simulink model "AEB_MODEL_F"  (R2022b)
settings: Solver=VariableStepAuto  StartTime=0.0  StopTime=10.0  RelTol=1e-3
model workspace (MAT data in the model file):
  DISTANCE = 100
  MASS_OF_THE_VEHICLE = 1500
  MIN_THRESHOLD_FOR_TTCmin = 0.7
  SPEED_OF_THE_EGO_VEHICLE = 80
  SPEED_OF_THE_LEADING_VEHICLE = 0
  TTC_EMERGE = 2
  Var = 0
libraries: simulink x37, spsOnDelayLib x1
(part 2 of 2)

== system AEB_MODEL_F/AEB/AEB_SYSTEM/FULL_BRAKE/FB_SYSTEM_IN_LOOP/CALCULATIONS_WITH_RESPECT_TO_TTC ==
  DISTANCE_TO_AVOID_COLLISION : Inport
  INITIAL_SPEED : Inport  Port=2
  TTC_FB_IN : Inport  Port=3
  CAL_BRAKING_DECCELERATION : Subsystem
      settings: RTWMemSecFuncInitTerm=Inherit_from_model  RTWMemSecFuncExecute=Inherit_from_model  RTWMemSecDataConstants=Inherit_from_model  RTWMemSecDataInternal=Inherit_from_model  RTWMemSecDataParameters=Inherit_from_model
  CAL_TTC : Subsystem
      settings: RTWMemSecFuncInitTerm=Inherit_from_model  RTWMemSecFuncExecute=Inherit_from_model  RTWMemSecDataConstants=Inherit_from_model  RTWMemSecDataInternal=Inherit_from_model  RTWMemSecDataParameters=Inherit_from_model
  CAL_inital_after_decceleration_speed : Subsystem
      settings: RTWMemSecFuncInitTerm=Inherit_from_model  RTWMemSecFuncExecute=Inherit_from_model  RTWMemSecDataConstants=Inherit_from_model  RTWMemSecDataInternal=Inherit_from_model  RTWMemSecDataParameters=Inherit_from_model
  CAL_remainig_distance : Subsystem
      settings: RTWMemSecFuncInitTerm=Inherit_from_model  RTWMemSecFuncExecute=Inherit_from_model  RTWMemSecDataConstants=Inherit_from_model  RTWMemSecDataInternal=Inherit_from_model  RTWMemSecDataParameters=Inherit_from_model
  Subsystem4 : Subsystem
      settings: RTWMemSecFuncInitTerm=Inherit_from_model  RTWMemSecFuncExecute=Inherit_from_model  RTWMemSecDataConstants=Inherit_from_model  RTWMemSecDataInternal=Inherit_from_model  RTWMemSecDataParameters=Inherit_from_model
  TTC_AFTER_FULL_BRAKE : Outport
  SPEED_AFTER_DECCELERATION : Outport  Port=2
  REMAINING_DISTANCE_FOR_NEXT_BRAKING_ : Outport  Port=3
  wires:
  INITIAL_SPEED/1 -> CAL_BRAKING_DECCELERATION/1(INITIAL_SPEED), CAL_inital_after_decceleration_speed/1(INITIAL_SPEED), CAL_remainig_distance/1(INITIAL_SPEED)  "INITIAL_SPEED"
  DISTANCE_TO_AVOID_COLLISION/1 -> CAL_BRAKING_DECCELERATION/2(REMAINING_DISTANCE_AFTER_PARTIAL_BRAKING), CAL_remainig_distance/2(DISTANCE_TO_AVOID_COLLISION)  "DISTANCE_TO_AVOID_COLLISION"
  CAL_inital_after_decceleration_speed/2(SPEED_AFTER_FB_DECCELERATION) -> SPEED_AFTER_DECCELERATION/1  "SPEED_AFTER_DECCELERATION"
  CAL_inital_after_decceleration_speed/1(INITIAL_SPEED_M/S) -> CAL_TTC/1(INITIAL_SPEED_M/S)
  CAL_TTC/1(TTC_AFTER_FULL_BRAKE) -> TTC_AFTER_FULL_BRAKE/1  "TTC_AFTER_FULL_BRAKE"
  CAL_remainig_distance/1(remainig_distance) -> REMAINING_DISTANCE_FOR_NEXT_BRAKING_/1, CAL_TTC/2(SPEED_AFTER_DECCELERATION)  "REMAINING_DISTANCE_FOR_NEXT_BRAKING_"
  CAL_BRAKING_DECCELERATION/1(FB_DECCELERATION) -> CAL_remainig_distance/4(FB_DECCELERATION), CAL_inital_after_decceleration_speed/3(FULL_BRAKING_DECCELERATION)  "FB_DECCELERATION"
  Subsystem4/1(TTC_FB_OUT) -> CAL_remainig_distance/3(TTC_FB), CAL_inital_after_decceleration_speed/2(TTC_FB)  "TTC_FB"
  TTC_FB_IN/1 -> Subsystem4/1(TTC_FB_IN)  "TTC_FB_IN"

== system AEB_MODEL_F/AEB/AEB_SYSTEM/FULL_BRAKE/FB_SYSTEM_IN_LOOP/REMAINING_DISTANCE ==
  REMAINING_DISTANCE_FOR_NEXT_BRAKING_ : Inport
  NEXT_ITERATION : Inport  Port=2
  Switch4 : Switch  Criteria=u2 > Threshold  SaturateOnIntegerOverflow=off  InputSameDT=off
  Unit_Delay4 : UnitDelay  SampleTime=-1  HasFrameUpgradeWarning=on
  RATE_OF_REMAINING_DISTANCE_FOR_NEXT_BRAKING_ : Outport
  CAL__REMAINING_DISTANCE_FOR_NEXT_BRAKING_ : Outport  Port=2
  wires:
  Unit_Delay4/1 -> Switch4/2, CAL__REMAINING_DISTANCE_FOR_NEXT_BRAKING_/1
  REMAINING_DISTANCE_FOR_NEXT_BRAKING_/1 -> Switch4/3
  Switch4/1 -> Unit_Delay4/1, RATE_OF_REMAINING_DISTANCE_FOR_NEXT_BRAKING_/1
  NEXT_ITERATION/1 -> Switch4/1

== system AEB_MODEL_F/AEB/AEB_SYSTEM/FULL_BRAKE/FB_SYSTEM_IN_LOOP/SPEED ==
  note: ego_and_leading_vehicle_speed_comparison
  SPEED_AFTER_FB_DECCELERATION : Inport
  NEXT_ITERATION : Inport  Port=2
  Compare_To_Constant : simulink/Logic and Bit Operations/Compare To Constant  relop=<=  const=SPEED_OF_THE_LEADING_VEHICLE  OutDataTypeStr=boolean
      settings: RTWMemSecFuncInitTerm=Inherit_from_model  RTWMemSecFuncExecute=Inherit_from_model  RTWMemSecDataConstants=Inherit_from_model  RTWMemSecDataInternal=Inherit_from_model  RTWMemSecDataParameters=Inherit_from_model
  Constant : Constant  Value=0
  Multiply : Gain  Gain=3.6
  Switch : Switch  Criteria=u2 > Threshold  SaturateOnIntegerOverflow=off  InputSameDT=off
  Switch4 : Switch  Criteria=u2 > Threshold  SaturateOnIntegerOverflow=off  InputSameDT=off
  Unit_Delay4 : UnitDelay  SampleTime=-1  HasFrameUpgradeWarning=on
  RATE_OF _SPEED : Outport
  CAL__SPEED_AFTER_DECCELERATION : Outport  Port=2
  tag scope: comp_speed_ego_and_leading3=global
  wires:
  SPEED_AFTER_FB_DECCELERATION/1 -> Switch4/3  "SPEED_AFTER_FB_DECCELERATION"
  NEXT_ITERATION/1 -> Switch4/1  "NEXT_ITERATION"
  Unit_Delay4/1 -> CAL__SPEED_AFTER_DECCELERATION/1, Switch4/2  "CAL__SPEED_AFTER_DECCELERATION"
  Switch/1 -> RATE_OF _SPEED/1  "RATE_OF _SPEED"
  Compare_To_Constant/1 -> [comp_speed_ego_and_leading3], Switch/2
  Multiply/1 -> Compare_To_Constant/1
  Constant/1 -> Switch/1
  Switch4/1 -> Unit_Delay4/1, Switch/3, Multiply/1

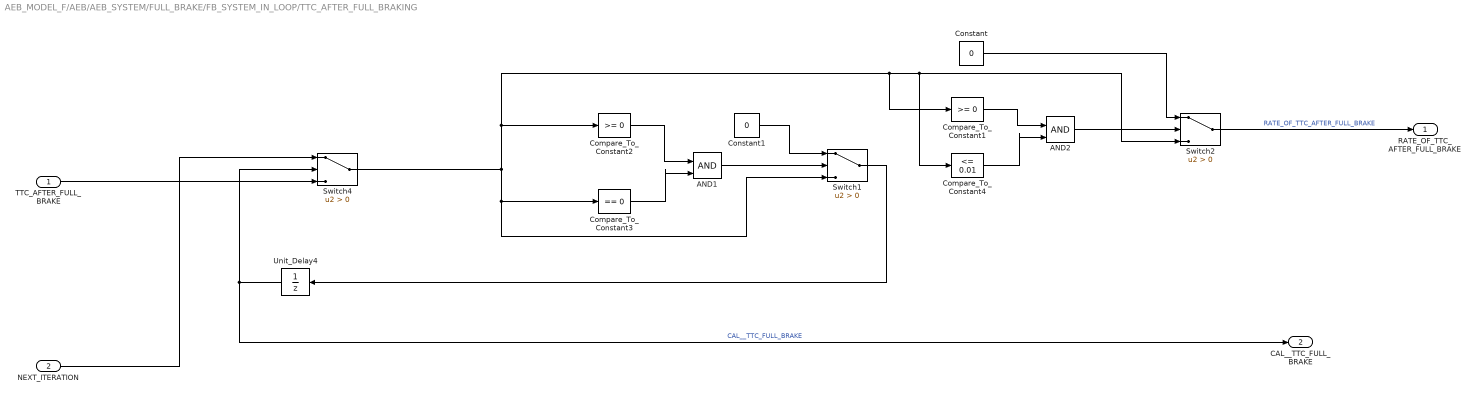
== system AEB_MODEL_F/AEB/AEB_SYSTEM/FULL_BRAKE/FB_SYSTEM_IN_LOOP/TTC_AFTER_FULL_BRAKING ==
  TTC_AFTER_FULL_BRAKE : Inport
  NEXT_ITERATION : Inport  Port=2
  AND1 : Logic  IconShape=distinctive  AllPortsSameDT=off  OutDataTypeStr=boolean
  AND2 : Logic  IconShape=distinctive  AllPortsSameDT=off  OutDataTypeStr=boolean
  Compare_To_Constant1 : simulink/Logic and Bit Operations/Compare To Constant  relop=>=  const=0  OutDataTypeStr=boolean
      settings: RTWMemSecFuncInitTerm=Inherit_from_model  RTWMemSecFuncExecute=Inherit_from_model  RTWMemSecDataConstants=Inherit_from_model  RTWMemSecDataInternal=Inherit_from_model  RTWMemSecDataParameters=Inherit_from_model
  Compare_To_Constant2 : simulink/Logic and Bit Operations/Compare To Constant  relop=>=  const=0  OutDataTypeStr=boolean
      settings: RTWMemSecFuncInitTerm=Inherit_from_model  RTWMemSecFuncExecute=Inherit_from_model  RTWMemSecDataConstants=Inherit_from_model  RTWMemSecDataInternal=Inherit_from_model  RTWMemSecDataParameters=Inherit_from_model
  Compare_To_Constant3 : simulink/Logic and Bit Operations/Compare To Constant  relop===  const=0  OutDataTypeStr=boolean
      settings: RTWMemSecFuncInitTerm=Inherit_from_model  RTWMemSecFuncExecute=Inherit_from_model  RTWMemSecDataConstants=Inherit_from_model  RTWMemSecDataInternal=Inherit_from_model  RTWMemSecDataParameters=Inherit_from_model
  Compare_To_Constant4 : simulink/Logic and Bit Operations/Compare To Constant  relop=<=  const=0.01  OutDataTypeStr=boolean
      settings: RTWMemSecFuncInitTerm=Inherit_from_model  RTWMemSecFuncExecute=Inherit_from_model  RTWMemSecDataConstants=Inherit_from_model  RTWMemSecDataInternal=Inherit_from_model  RTWMemSecDataParameters=Inherit_from_model
  Constant : Constant  Value=0
  Constant1 : Constant  Value=0
  Switch1 : Switch  Criteria=u2 > Threshold  SaturateOnIntegerOverflow=off  InputSameDT=off
  Switch2 : Switch  Criteria=u2 > Threshold  SaturateOnIntegerOverflow=off  InputSameDT=off
  Switch4 : Switch  Criteria=u2 > Threshold  SaturateOnIntegerOverflow=off  InputSameDT=off
  Unit_Delay4 : UnitDelay  SampleTime=-1  HasFrameUpgradeWarning=on
  RATE_OF_TTC_AFTER_FULL_BRAKE : Outport
  CAL__TTC_FULL_BRAKE : Outport  Port=2
  wires:
  Unit_Delay4/1 -> Switch4/2, CAL__TTC_FULL_BRAKE/1  "CAL__TTC_FULL_BRAKE"
  TTC_AFTER_FULL_BRAKE/1 -> Switch4/3
  NEXT_ITERATION/1 -> Switch4/1
  Compare_To_Constant2/1 -> AND1/1
  Compare_To_Constant3/1 -> AND1/2
  AND1/1 -> Switch1/2
  Switch1/1 -> Unit_Delay4/1
  Constant1/1 -> Switch1/1
  Switch2/1 -> RATE_OF_TTC_AFTER_FULL_BRAKE/1  "RATE_OF_TTC_AFTER_FULL_BRAKE"
  Switch4/1 -> Compare_To_Constant1/1, Switch2/3, Compare_To_Constant4/1, Compare_To_Constant2/1, Switch1/3, Compare_To_Constant3/1
  AND2/1 -> Switch2/2
  Constant/1 -> Switch2/1
  Compare_To_Constant1/1 -> AND2/1
  Compare_To_Constant4/1 -> AND2/2

== system AEB_MODEL_F/AEB/AEB_SYSTEM/PARTIAL_BRAKE/PARTIAL_BRAKING/PB_CALCULATIONS ==
  note: ego_and_leading_vehicle_speed_comparison
  note: CAL_PB
  DISTANCE_TO_AVOID_COLLISION : Inport
  INITIAL_SPEED : Inport  Port=2
  TTCmin : Inport  Port=3
  CAL_BRAKING_DECCELERATION : Subsystem
      settings: RTWMemSecFuncInitTerm=Inherit_from_model  RTWMemSecFuncExecute=Inherit_from_model  RTWMemSecDataConstants=Inherit_from_model  RTWMemSecDataInternal=Inherit_from_model  RTWMemSecDataParameters=Inherit_from_model
  CAL_INITAL_AFTER_DECCELERATION_SPEED : Subsystem
      settings: RTWMemSecFuncInitTerm=Inherit_from_model  RTWMemSecFuncExecute=Inherit_from_model  RTWMemSecDataConstants=Inherit_from_model  RTWMemSecDataInternal=Inherit_from_model  RTWMemSecDataParameters=Inherit_from_model
  CAL_REMAINING_DISTANCE : Subsystem
      settings: RTWMemSecFuncInitTerm=Inherit_from_model  RTWMemSecFuncExecute=Inherit_from_model  RTWMemSecDataConstants=Inherit_from_model  RTWMemSecDataInternal=Inherit_from_model  RTWMemSecDataParameters=Inherit_from_model
  CAL_TTC : Subsystem
      settings: RTWMemSecFuncInitTerm=Inherit_from_model  RTWMemSecFuncExecute=Inherit_from_model  RTWMemSecDataConstants=Inherit_from_model  RTWMemSecDataInternal=Inherit_from_model  RTWMemSecDataParameters=Inherit_from_model
  Compare_To_Constant : simulink/Logic and Bit Operations/Compare To Constant  relop=<=  const=SPEED_OF_THE_LEADING_VEHICLE  OutDataTypeStr=boolean
      settings: RTWMemSecFuncInitTerm=Inherit_from_model  RTWMemSecFuncExecute=Inherit_from_model  RTWMemSecDataConstants=Inherit_from_model  RTWMemSecDataInternal=Inherit_from_model  RTWMemSecDataParameters=Inherit_from_model
  Constant : Constant  Value=0
  Switch : Switch  Criteria=u2 > Threshold  SaturateOnIntegerOverflow=off  InputSameDT=off
  m/s_to_km/s : Gain  Gain=3.6
  TTC_AFTER_PARTITAL_BRAKE : Outport
  SPEED_AFTER_PB_DECCELERATION : Outport  Port=2
  REMAINING_DISTANCE_FOR_NEXT_BRAKING : Outport  Port=3
  tag scope: comp_speed_ego_and_leading_PB=global
  wires:
  CAL_BRAKING_DECCELERATION/1(PB_DECCELERATION) -> CAL_INITAL_AFTER_DECCELERATION_SPEED/3(PARTIAL_BRAKING_DECCELERATION), CAL_REMAINING_DISTANCE/4(PB_DECCELERATION)  "PB_DECCELERATION"
  INITIAL_SPEED/1 -> CAL_REMAINING_DISTANCE/1(INITIAL_SPEED), CAL_INITAL_AFTER_DECCELERATION_SPEED/1(INITIAL_SPEED)  "INITIAL_SPEED"
  TTCmin/1 -> CAL_INITAL_AFTER_DECCELERATION_SPEED/2(TTC_PB), CAL_REMAINING_DISTANCE/3(TTC_PB)  "TTCmin"
  CAL_INITAL_AFTER_DECCELERATION_SPEED/1(INITIAL_SPEED_M/S) -> CAL_TTC/1(INITIAL_SPEED_M/S)
  DISTANCE_TO_AVOID_COLLISION/1 -> CAL_BRAKING_DECCELERATION/1(DISTANCE_TO_AVOID_COLLISION), CAL_REMAINING_DISTANCE/2(DISTANCE_TO_AVOID_COLLISION)  "DISTANCE_TO_AVOID_COLLISION"
  CAL_INITAL_AFTER_DECCELERATION_SPEED/2(SPEED_AFTER_PB_DECCELERATION) -> m/s_to_km/s/1, Switch/3
  CAL_TTC/1(TTC_AFTER_PARTITAL_BRAKE) -> TTC_AFTER_PARTITAL_BRAKE/1  "TTC_AFTER_PARTITAL_BRAKE"
  CAL_REMAINING_DISTANCE/1(REMAINING_DISTANCE) -> CAL_TTC/2(SPEED_AFTER_PB_DECCELERATION), REMAINING_DISTANCE_FOR_NEXT_BRAKING/1  "REMAINING_DISTANCE_FOR_NEXT_BRAKING"
  m/s_to_km/s/1 -> Compare_To_Constant/1
  Compare_To_Constant/1 -> Switch/2, [comp_speed_ego_and_leading_PB]
  Constant/1 -> Switch/1
  Switch/1 -> SPEED_AFTER_PB_DECCELERATION/1  "SPEED_AFTER_PB_DECCELERATION"

== system AEB_MODEL_F/AEB/AEB_SYSTEM/PARTIAL_BRAKE/PARTIAL_BRAKING/PB_IN_LOOP ==
  note: condt_distance_travelled_after_brake
  TTC_AFTER_PARTITAL_BRAKE : Inport
  _SPEED_AFTER_PB_DECCELERATION : Inport  Port=2
  REMAINING_DISTANCE_FOR_NEXT_BRAKING_ : Inport  Port=3
  CALCULATIONS_WITH_RESPECT_TO_TTC : Subsystem
      settings: RTWMemSecFuncInitTerm=Inherit_from_model  RTWMemSecFuncExecute=Inherit_from_model  RTWMemSecDataConstants=Inherit_from_model  RTWMemSecDataInternal=Inherit_from_model  RTWMemSecDataParameters=Inherit_from_model
  Constant : Constant  Value=0
  REMAINING_DISTANCE : Subsystem
      settings: RTWMemSecFuncInitTerm=Inherit_from_model  RTWMemSecFuncExecute=Inherit_from_model  RTWMemSecDataConstants=Inherit_from_model  RTWMemSecDataInternal=Inherit_from_model  RTWMemSecDataParameters=Inherit_from_model
  SPEED : Subsystem
      settings: RTWMemSecFuncInitTerm=Inherit_from_model  RTWMemSecFuncExecute=Inherit_from_model  RTWMemSecDataConstants=Inherit_from_model  RTWMemSecDataInternal=Inherit_from_model  RTWMemSecDataParameters=Inherit_from_model
  Subtract : Sum  Inputs=+-
  Switch : Switch  Criteria=u2 > Threshold  SaturateOnIntegerOverflow=off  InputSameDT=off
  TTC_AFTER_PARTIAL_BRAKING : Subsystem
      settings: RTWMemSecFuncInitTerm=Inherit_from_model  RTWMemSecFuncExecute=Inherit_from_model  RTWMemSecDataConstants=Inherit_from_model  RTWMemSecDataInternal=Inherit_from_model  RTWMemSecDataParameters=Inherit_from_model
  RATE_OF_ TTC_AFTER_PARTITAL_BRAKE : Outport
  RATE_OF_SPEED : Outport  Port=2
  RATE_OF _REMAINING_DISTANCE_FOR_NEXT_BRAKING_ : Outport  Port=3
  wires:
  CALCULATIONS_WITH_RESPECT_TO_TTC/2(SPEED_AFTER_PB_DECCELERATION) -> SPEED/2(NEXT_ITERATION)  "SPEED_AFTER_PB_DECCELERATION"
  REMAINING_DISTANCE/1(RATE_OF_REMAINING_DISTANCE_FOR_NEXT_BRAKING_) -> Subtract/2, Switch/2, RATE_OF _REMAINING_DISTANCE_FOR_NEXT_BRAKING_/1  "RATE_OF _REMAINING_DISTANCE_FOR_NEXT_BRAKING_"
  CALCULATIONS_WITH_RESPECT_TO_TTC/3(REMAINING_DISTANCE_FOR_NEXT_BRAKING_) -> REMAINING_DISTANCE/2(NEXT_ITERATION)  "REMAINING_DISTANCE_FOR_NEXT_BRAKING_"
  REMAINING_DISTANCE/2(CAL__REMAINING_DISTANCE_FOR_NEXT_BRAKING_) -> CALCULATIONS_WITH_RESPECT_TO_TTC/1(DISTANCE_TO_AVOID_COLLISION)  "CAL__REMAINING_DISTANCE_FOR_NEXT_BRAKING_"
  SPEED/2(CAL__SPEED_AFTER_PB_DECCELERATION) -> CALCULATIONS_WITH_RESPECT_TO_TTC/2(INITIAL_SPEED)  "CAL__SPEED_AFTER_PB_DECCELERATION"
  SPEED/1(RATE_OF_SPEED) -> RATE_OF_SPEED/1  "RATE_OF_SPEED"
  _SPEED_AFTER_PB_DECCELERATION/1 -> SPEED/1(SPEED_AFTER_PARTITAL_BRAKE_)  "_SPEED_AFTER_PB_DECCELERATION"
  REMAINING_DISTANCE_FOR_NEXT_BRAKING_/1 -> REMAINING_DISTANCE/1(REMAINING_DISTANCE_FOR_NEXT_BRAKING _)  "REMAINING_DISTANCE_FOR_NEXT_BRAKING_"
  TTC_AFTER_PARTIAL_BRAKING/2(CAL__TTCmin) -> CALCULATIONS_WITH_RESPECT_TO_TTC/3(TTC_PB_IN)  "CAL__TTCmin"
  CALCULATIONS_WITH_RESPECT_TO_TTC/1(TTC_AFTER_PARTITAL_BRAKE) -> TTC_AFTER_PARTIAL_BRAKING/2(NEXT_ITERATION)  "TTC_AFTER_PARTITAL_BRAKE"
  TTC_AFTER_PARTITAL_BRAKE/1 -> TTC_AFTER_PARTIAL_BRAKING/1(TTC_AFTER_PARTITAL_BRAKE)  "TTC_AFTER_PARTITAL_BRAKE"
  Constant/1 -> Switch/3
  TTC_AFTER_PARTIAL_BRAKING/1(RATE_OF_TTC_AFTER_PARTITAL_BRAKE) -> RATE_OF_ TTC_AFTER_PARTITAL_BRAKE/1  "RATE_OF_ TTC_AFTER_PARTITAL_BRAKE"
  Subtract/1 -> Switch/1
  [DISTANCE_TO_AVOID_COLLISION] -> Subtract/1
  Switch/1 -> ?  "PARTIAL_BRAKE_DISTANCE_TRAVELLED_"

== system AEB_MODEL_F/AEB/BRAKE_PEDAL_FORCE_and_DIAGNOSTIC_CHECKS/BRAKE_PEDAL_FORCE_CALCULATION/COMPARING_THE_BOTH_BRAKING_DECCELERATION_VALUES/CAL.KM//Hr_TO_M//Hr_and_DISTANCE_TO_AVOID_COLLISION ==
  note: CONDITION_FOR_CHECKING_REACTION_TIME
  note: condt_TTC>5;_AEB_OFF
  INITIAL_SPEED : Inport
  DISTANCE : Inport  Port=2
  CAL_TTC : Constant  Value=DISTANCE/(SPEED_OF_THE_EGO_VEHICLE-SPEED_OF_THE_LEADING_VEHICLE)*3.6
  Compare_To_Constant : simulink/Logic and Bit Operations/Compare To Constant  relop=<  const=5  OutDataTypeStr=boolean
      settings: RTWMemSecFuncInitTerm=Inherit_from_model  RTWMemSecFuncExecute=Inherit_from_model  RTWMemSecDataConstants=Inherit_from_model  RTWMemSecDataInternal=Inherit_from_model  RTWMemSecDataParameters=Inherit_from_model
  Constant : Constant  Value=0
  Constant1 : Constant
  Divide : Product  Inputs=*/
  KM/HR_TO_M/S : Constant  Value=3.6
  Subtract : Sum  Inputs=+-
  Subtract1 : Sum  Inputs=+-
  Switch : Switch  Criteria=u2 > Threshold  SaturateOnIntegerOverflow=off  InputSameDT=off
  INITIAL_SPEED_M/S : Outport
  DISTANCE_TO_AVOID_COLLISION : Outport  Port=2
  wires:
  Subtract/1 -> Subtract1/1  "REACTION_DISTANCE"
  Constant1/1 -> Subtract1/2
  Divide/1 -> INITIAL_SPEED_M/S/1, Switch/3  "INITIAL_SPEED_M/S"
  Switch/1 -> Subtract/2  "condt_TTC<5"
  Subtract1/1 -> DISTANCE_TO_AVOID_COLLISION/1  "DISTANCE_TO_AVOID_COLLISION"
  INITIAL_SPEED/1 -> Divide/1  "SPEED"
  DISTANCE/1 -> Subtract/1  "DISTANCE"
  Compare_To_Constant/1 -> Switch/2
  KM/HR_TO_M/S/1 -> Divide/2
  CAL_TTC/1 -> Compare_To_Constant/1  "CAL_TTC"
  Constant/1 -> Switch/1

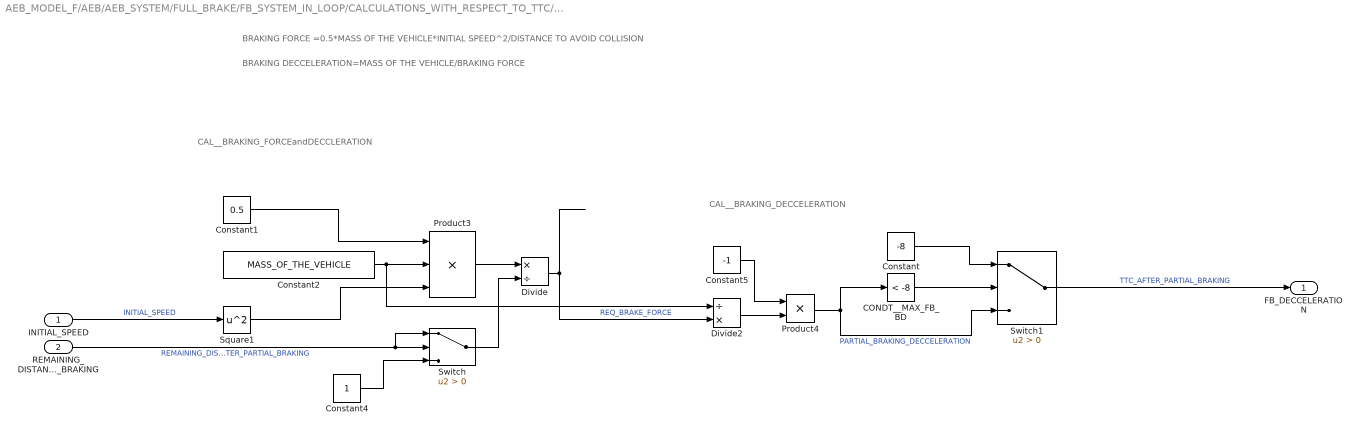
== system AEB_MODEL_F/AEB/AEB_SYSTEM/FULL_BRAKE/FB_SYSTEM_IN_LOOP/CALCULATIONS_WITH_RESPECT_TO_TTC/CAL_BRAKING_DECCELERATION ==
  note: BRAKING DECCELERATION=MASS OF THE VEHICLE/BRAKING FORCE
  note: BRAKING FORCE =0.5*MASS OF THE VEHICLE*INITIAL SPEED^2/DISTANCE TO AVOID COLLISION
  note: CAL__BRAKING_DECCELERATION
  note: CAL__BRAKING_FORCEandDECCLERATION
  INITIAL_SPEED : Inport
  REMAINING_DISTANCE_AFTER_PARTIAL_BRAKING : Inport  Port=2
  CONDT__MAX_FB_BD : simulink/Logic and Bit Operations/Compare To Constant  relop=<  const=-8  OutDataTypeStr=boolean
      settings: RTWMemSecFuncInitTerm=Inherit_from_model  RTWMemSecFuncExecute=Inherit_from_model  RTWMemSecDataConstants=Inherit_from_model  RTWMemSecDataInternal=Inherit_from_model  RTWMemSecDataParameters=Inherit_from_model
  Constant : Constant  Value=-8
  Constant1 : Constant  Value=0.5
  Constant2 : Constant  Value=MASS_OF_THE_VEHICLE
  Constant4 : Constant
  Constant5 : Constant  Value=-1
  Divide : Product  Inputs=*/
  Divide2 : Product  Inputs=/*
  Product3 : Product  Inputs=3
  Product4 : Product
  Square1 : Math  Operator=square
  Switch : Switch  Criteria=u2 > Threshold  SaturateOnIntegerOverflow=off  InputSameDT=off
  Switch1 : Switch  Criteria=u2 > Threshold  SaturateOnIntegerOverflow=off  InputSameDT=off
  FB_DECCELERATION : Outport
  wires:
  CONDT__MAX_FB_BD/1 -> Switch1/2
  Constant/1 -> Switch1/1
  INITIAL_SPEED/1 -> Square1/1  "INITIAL_SPEED"
  Constant4/1 -> Switch/3
  Switch/1 -> Divide/2
  Divide2/1 -> Product4/2
  Constant2/1 -> Divide2/1, Product3/2
  Product3/1 -> Divide/1
  REMAINING_DISTANCE_AFTER_PARTIAL_BRAKING/1 -> Switch/1, Switch/2  "REMAINING_DISTANCE_AFTER_PARTIAL_BRAKING"
  Constant5/1 -> Product4/1
  Switch1/1 -> FB_DECCELERATION/1  "TTC_AFTER_PARTIAL_BRAKING"
  Square1/1 -> Product3/3
  Product4/1 -> Switch1/3, CONDT__MAX_FB_BD/1  "PARTIAL_BRAKING_DECCELERATION"
  Divide/1 -> Divide2/2  "REQ_BRAKE_FORCE"
  Constant1/1 -> Product3/1

== system AEB_MODEL_F/AEB/AEB_SYSTEM/FULL_BRAKE/FB_SYSTEM_IN_LOOP/CALCULATIONS_WITH_RESPECT_TO_TTC/CAL_TTC ==
  INITIAL_SPEED_M/S : Inport
  SPEED_AFTER_DECCELERATION : Inport  Port=2
  Constant6 : Constant
  Divide1 : Product  Inputs=/*
  Switch2 : Switch  Criteria=u2 > Threshold  SaturateOnIntegerOverflow=off  InputSameDT=off
  TTC_AFTER_FULL_BRAKE : Outport
  wires:
  Constant6/1 -> Switch2/3
  Switch2/1 -> Divide1/1
  INITIAL_SPEED_M/S/1 -> Switch2/2, Switch2/1  "INITIAL_SPEED_M/S"
  SPEED_AFTER_DECCELERATION/1 -> Divide1/2  "SPEED_AFTER_DECCELERATION"
  Divide1/1 -> TTC_AFTER_FULL_BRAKE/1  "TTC_AFTER_FULL_BRAKE"

== system AEB_MODEL_F/AEB/AEB_SYSTEM/FULL_BRAKE/FB_SYSTEM_IN_LOOP/CALCULATIONS_WITH_RESPECT_TO_TTC/CAL_inital_after_decceleration_speed ==
  note: Speed after deceleration:
      | V = u + at
  INITIAL_SPEED : Inport
  TTC_FB : Inport  Port=2
  FULL_BRAKING_DECCELERATION : Inport  Port=3
  Product5 : Product
  Subtract1 : Sum
  INITIAL_SPEED_M/S : Outport
  SPEED_AFTER_FB_DECCELERATION : Outport  Port=2
  wires:
  INITIAL_SPEED/1 -> Subtract1/1  "INITIAL_SPEED"
  FULL_BRAKING_DECCELERATION/1 -> Product5/1  "FULL_BRAKING_DECCELERATION"
  Product5/1 -> Subtract1/2
  Subtract1/1 -> SPEED_AFTER_FB_DECCELERATION/1, INITIAL_SPEED_M/S/1  "INITIAL_SPEED_M/S"
  TTC_FB/1 -> Product5/2  "TTC_FB"

== system AEB_MODEL_F/AEB/AEB_SYSTEM/FULL_BRAKE/FB_SYSTEM_IN_LOOP/CALCULATIONS_WITH_RESPECT_TO_TTC/CAL_remainig_distance ==
  note: Remaining distance= ut + 1/2(at^2)
  INITIAL_SPEED : Inport
  DISTANCE_TO_AVOID_COLLISION : Inport  Port=2
  TTC_FB : Inport  Port=3
  FB_DECCELERATION : Inport  Port=4
  Add1 : Sum
  Constant3 : Constant  Value=0.5
  Product1 : Product  Inputs=3
  Product2 : Product
  Square2 : Math  Operator=square
  Subtract3 : Sum  Inputs=+-
  remainig_distance : Outport
  wires:
  Add1/1 -> Subtract3/2
  TTC_FB/1 -> Square2/1, Product2/2  "TTC_FB"
  Square2/1 -> Product1/3
  Subtract3/1 -> remainig_distance/1  "remainig_distance"
  Product1/1 -> Add1/2
  Product2/1 -> Add1/1
  Constant3/1 -> Product1/1
  FB_DECCELERATION/1 -> Product1/2  "FB_DECCELERATION"
  DISTANCE_TO_AVOID_COLLISION/1 -> Subtract3/1  "DISTANCE_TO_AVOID_COLLISION"
  INITIAL_SPEED/1 -> Product2/1  "INITIAL_SPEED"

== system AEB_MODEL_F/AEB/AEB_SYSTEM/FULL_BRAKE/FB_SYSTEM_IN_LOOP/CALCULATIONS_WITH_RESPECT_TO_TTC/Subsystem4 ==
  TTC_FB_IN : Inport
  AND1 : Logic  IconShape=distinctive  AllPortsSameDT=off  OutDataTypeStr=boolean
  Compare_To_Constant2 : simulink/Logic and Bit Operations/Compare To Constant  relop=<=  const=0.03  OutDataTypeStr=boolean
      settings: RTWMemSecFuncInitTerm=Inherit_from_model  RTWMemSecFuncExecute=Inherit_from_model  RTWMemSecDataConstants=Inherit_from_model  RTWMemSecDataInternal=Inherit_from_model  RTWMemSecDataParameters=Inherit_from_model
  Compare_To_Constant3 : simulink/Logic and Bit Operations/Compare To Constant  relop=>  const=0  OutDataTypeStr=boolean
      settings: RTWMemSecFuncInitTerm=Inherit_from_model  RTWMemSecFuncExecute=Inherit_from_model  RTWMemSecDataConstants=Inherit_from_model  RTWMemSecDataInternal=Inherit_from_model  RTWMemSecDataParameters=Inherit_from_model
  Constant : Constant  Value=0
  Switch1 : Switch  Criteria=u2 > Threshold  SaturateOnIntegerOverflow=off  InputSameDT=off
  TTC_FB_OUT : Outport
  wires:
  AND1/1 -> Switch1/2
  Compare_To_Constant3/1 -> AND1/2
  Compare_To_Constant2/1 -> AND1/1
  TTC_FB_IN/1 -> Compare_To_Constant2/1, Switch1/3, Compare_To_Constant3/1
  Switch1/1 -> TTC_FB_OUT/1
  Constant/1 -> Switch1/1

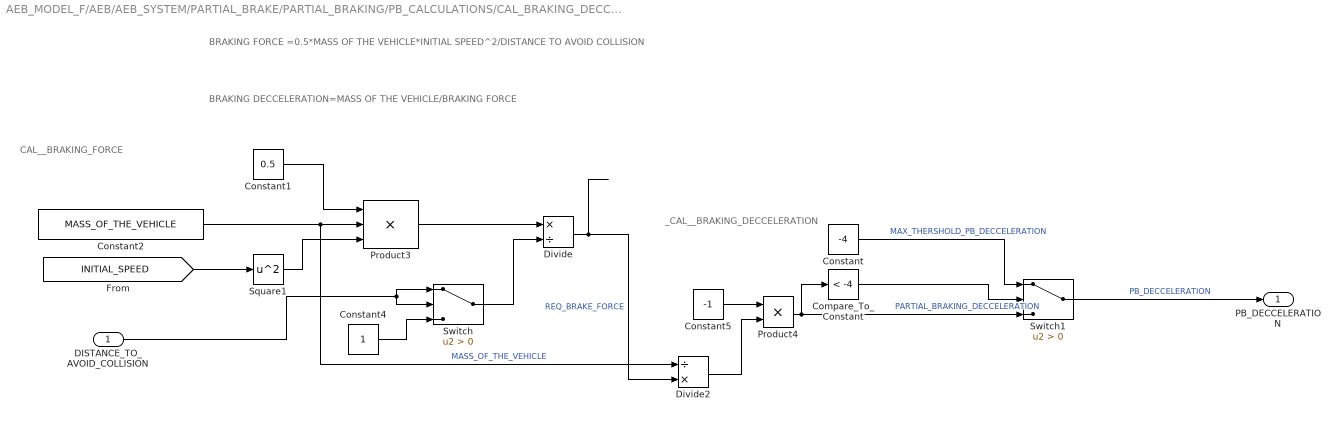
== system AEB_MODEL_F/AEB/AEB_SYSTEM/PARTIAL_BRAKE/PARTIAL_BRAKING/PB_CALCULATIONS/CAL_BRAKING_DECCELERATION ==
  note: _CAL__BRAKING_DECCELERATION
  note: CAL__BRAKING_FORCE
  note: BRAKING FORCE =0.5*MASS OF THE VEHICLE*INITIAL SPEED^2/DISTANCE TO AVOID COLLISION
  note: BRAKING DECCELERATION=MASS OF THE VEHICLE/BRAKING FORCE
  DISTANCE_TO_AVOID_COLLISION : Inport
  Compare_To_Constant : simulink/Logic and Bit Operations/Compare To Constant  relop=<  const=-4  OutDataTypeStr=boolean
      settings: RTWMemSecFuncInitTerm=Inherit_from_model  RTWMemSecFuncExecute=Inherit_from_model  RTWMemSecDataConstants=Inherit_from_model  RTWMemSecDataInternal=Inherit_from_model  RTWMemSecDataParameters=Inherit_from_model
  Constant : Constant  Value=-4
  Constant1 : Constant  Value=0.5
  Constant2 : Constant  Value=MASS_OF_THE_VEHICLE
  Constant4 : Constant
  Constant5 : Constant  Value=-1
  Divide : Product  Inputs=*/
  Divide2 : Product  Inputs=/*
  Product3 : Product  Inputs=3
  Product4 : Product
  Square1 : Math  Operator=square
  Switch : Switch  Criteria=u2 > Threshold  SaturateOnIntegerOverflow=off  InputSameDT=off
  Switch1 : Switch  Criteria=u2 > Threshold  SaturateOnIntegerOverflow=off  InputSameDT=off
  PB_DECCELERATION : Outport
  wires:
  DISTANCE_TO_AVOID_COLLISION/1 -> Switch/2, Switch/1
  Divide2/1 -> Product4/2
  Constant2/1 -> Divide2/1, Product3/2  "MASS_OF_THE_VEHICLE"
  Product4/1 -> Switch1/3, Compare_To_Constant/1  "PARTIAL_BRAKING_DECCELERATION"
  Constant1/1 -> Product3/1
  Divide/1 -> Divide2/2  "REQ_BRAKE_FORCE"
  Constant4/1 -> Switch/3
  Square1/1 -> Product3/3
  Product3/1 -> Divide/1
  Switch/1 -> Divide/2
  [INITIAL_SPEED] -> Square1/1
  Constant5/1 -> Product4/1
  Constant/1 -> Switch1/1  "MAX_THERSHOLD_PB_DECCELERATION"
  Switch1/1 -> PB_DECCELERATION/1  "PB_DECCELERATION"
  Compare_To_Constant/1 -> Switch1/2

== system AEB_MODEL_F/AEB/AEB_SYSTEM/PARTIAL_BRAKE/PARTIAL_BRAKING/PB_CALCULATIONS/CAL_INITAL_AFTER_DECCELERATION_SPEED ==
  note: Speed after deceleration:
      | V = u + at
  INITIAL_SPEED : Inport
  TTC_PB : Inport  Port=2
  PARTIAL_BRAKING_DECCELERATION : Inport  Port=3
  Product5 : Product
  Subtract1 : Sum
  INITIAL_SPEED_M/S : Outport
  SPEED_AFTER_PB_DECCELERATION : Outport  Port=2
  wires:
  INITIAL_SPEED/1 -> Subtract1/1  "INITIAL_SPEED"
  PARTIAL_BRAKING_DECCELERATION/1 -> Product5/1  "PARTIAL_BRAKING_DECCELERATION"
  Product5/1 -> Subtract1/2
  Subtract1/1 -> SPEED_AFTER_PB_DECCELERATION/1, INITIAL_SPEED_M/S/1  "INITIAL_SPEED_M/S"
  TTC_PB/1 -> Product5/2  "TTC_PB"

== system AEB_MODEL_F/AEB/AEB_SYSTEM/PARTIAL_BRAKE/PARTIAL_BRAKING/PB_CALCULATIONS/CAL_REMAINING_DISTANCE ==
  note: Remaining distance= ut + 1/2(at^2)
  INITIAL_SPEED : Inport
  DISTANCE_TO_AVOID_COLLISION : Inport  Port=2
  TTC_PB : Inport  Port=3
  PB_DECCELERATION : Inport  Port=4
  Add1 : Sum
  Constant3 : Constant  Value=0.5
  Product1 : Product  Inputs=3
  Product2 : Product
  Square2 : Math  Operator=square
  Subtract3 : Sum  Inputs=+-
  REMAINING_DISTANCE : Outport
  wires:
  Add1/1 -> Subtract3/2
  TTC_PB/1 -> Square2/1, Product2/2  "TTC_PB"
  Square2/1 -> Product1/3
  Subtract3/1 -> REMAINING_DISTANCE/1  "REMAINING_DISTANCE"
  Product1/1 -> Add1/2
  Product2/1 -> Add1/1
  Constant3/1 -> Product1/1
  PB_DECCELERATION/1 -> Product1/2  "PB_DECCELERATION"
  DISTANCE_TO_AVOID_COLLISION/1 -> Subtract3/1  "DISTANCE_TO_AVOID_COLLISION"
  INITIAL_SPEED/1 -> Product2/1  "INITIAL_SPEED"

== system AEB_MODEL_F/AEB/AEB_SYSTEM/PARTIAL_BRAKE/PARTIAL_BRAKING/PB_CALCULATIONS/CAL_TTC ==
  INITIAL_SPEED_M/S : Inport
  SPEED_AFTER_PB_DECCELERATION : Inport  Port=2
  Constant6 : Constant
  Divide1 : Product  Inputs=/*
  Switch2 : Switch  Criteria=u2 > Threshold  SaturateOnIntegerOverflow=off  InputSameDT=off
  TTC_AFTER_PARTITAL_BRAKE : Outport
  wires:
  Constant6/1 -> Switch2/3
  Switch2/1 -> Divide1/1
  INITIAL_SPEED_M/S/1 -> Switch2/2, Switch2/1  "INITIAL_SPEED_M/S"
  SPEED_AFTER_PB_DECCELERATION/1 -> Divide1/2  "SPEED_AFTER_PB_DECCELERATION"
  Divide1/1 -> TTC_AFTER_PARTITAL_BRAKE/1  "TTC_AFTER_PARTITAL_BRAKE"

== system AEB_MODEL_F/AEB/AEB_SYSTEM/PARTIAL_BRAKE/PARTIAL_BRAKING/PB_IN_LOOP/CALCULATIONS_WITH_RESPECT_TO_TTC ==
  DISTANCE_TO_AVOID_COLLISION : Inport
  INITIAL_SPEED : Inport  Port=2
  TTC_PB_IN : Inport  Port=3
  CAL_BRAKING_DECCELERATION : Subsystem
      settings: RTWMemSecFuncInitTerm=Inherit_from_model  RTWMemSecFuncExecute=Inherit_from_model  RTWMemSecDataConstants=Inherit_from_model  RTWMemSecDataInternal=Inherit_from_model  RTWMemSecDataParameters=Inherit_from_model
  CAL_TTC : Subsystem
      settings: RTWMemSecFuncInitTerm=Inherit_from_model  RTWMemSecFuncExecute=Inherit_from_model  RTWMemSecDataConstants=Inherit_from_model  RTWMemSecDataInternal=Inherit_from_model  RTWMemSecDataParameters=Inherit_from_model
  CAL_inital_after_decceleration_speed : Subsystem
      settings: RTWMemSecFuncInitTerm=Inherit_from_model  RTWMemSecFuncExecute=Inherit_from_model  RTWMemSecDataConstants=Inherit_from_model  RTWMemSecDataInternal=Inherit_from_model  RTWMemSecDataParameters=Inherit_from_model
  CAL_remainig_distance : Subsystem
      settings: RTWMemSecFuncInitTerm=Inherit_from_model  RTWMemSecFuncExecute=Inherit_from_model  RTWMemSecDataConstants=Inherit_from_model  RTWMemSecDataInternal=Inherit_from_model  RTWMemSecDataParameters=Inherit_from_model
  TTC_LIMIT : Subsystem
      settings: RTWMemSecFuncInitTerm=Inherit_from_model  RTWMemSecFuncExecute=Inherit_from_model  RTWMemSecDataConstants=Inherit_from_model  RTWMemSecDataInternal=Inherit_from_model  RTWMemSecDataParameters=Inherit_from_model
  TTC_AFTER_PARTITAL_BRAKE : Outport
  SPEED_AFTER_PB_DECCELERATION : Outport  Port=2
  REMAINING_DISTANCE_FOR_NEXT_BRAKING_ : Outport  Port=3
  wires:
  INITIAL_SPEED/1 -> CAL_BRAKING_DECCELERATION/1(INITIAL_SPEED), CAL_inital_after_decceleration_speed/1(INITIAL_SPEED), CAL_remainig_distance/1(INITIAL_SPEED)  "INITIAL_SPEED"
  DISTANCE_TO_AVOID_COLLISION/1 -> CAL_BRAKING_DECCELERATION/2(DISTANCE_TO_AVOID_COLLISION), CAL_remainig_distance/2(DISTANCE_TO_AVOID_COLLISION)  "DISTANCE_TO_AVOID_COLLISION"
  CAL_inital_after_decceleration_speed/2(SPEED_AFTER_PB_DECCELERATION) -> SPEED_AFTER_PB_DECCELERATION/1  "SPEED_AFTER_PB_DECCELERATION"
  CAL_inital_after_decceleration_speed/1(INITIAL_SPEED_M/S) -> CAL_TTC/1(INITIAL_SPEED_M/S)  "INITIAL_SPEED"
  CAL_TTC/1(TTC_AFTER_PARTITAL_BRAKE) -> TTC_AFTER_PARTITAL_BRAKE/1  "TTC_AFTER_PARTITAL_BRAKE"
  CAL_remainig_distance/1(Remainig_distance) -> CAL_TTC/2(SPEED_AFTER_PB_DECCELERATION), REMAINING_DISTANCE_FOR_NEXT_BRAKING_/1  "Remainig_distance"
  CAL_BRAKING_DECCELERATION/1(PB_DECCELERATION) -> CAL_remainig_distance/4(PB_DECCELERATION), CAL_inital_after_decceleration_speed/3(PARTIAL_BRAKING_DECCELERATION)  "PB_DECCELERATION"
  TTC_LIMIT/1(TTC_PB) -> CAL_inital_after_decceleration_speed/2(TTC_PB), CAL_remainig_distance/3(TTC_PB)  "TTC_PB"
  TTC_PB_IN/1 -> TTC_LIMIT/1(TTC_PB_)  "TTC_PB_IN"

== system AEB_MODEL_F/AEB/AEB_SYSTEM/PARTIAL_BRAKE/PARTIAL_BRAKING/PB_IN_LOOP/REMAINING_DISTANCE ==
  REMAINING_DISTANCE_FOR_NEXT_BRAKING _ : Inport
  NEXT_ITERATION : Inport  Port=2
  Switch4 : Switch  Criteria=u2 > Threshold  SaturateOnIntegerOverflow=off  InputSameDT=off
  Unit_Delay4 : UnitDelay  SampleTime=-1  HasFrameUpgradeWarning=on
  RATE_OF_REMAINING_DISTANCE_FOR_NEXT_BRAKING_ : Outport
  CAL__REMAINING_DISTANCE_FOR_NEXT_BRAKING_ : Outport  Port=2
  wires:
  REMAINING_DISTANCE_FOR_NEXT_BRAKING _/1 -> Switch4/3  "REMAINING_DISTANCE_FOR_NEXT_BRAKING _"
  Switch4/1 -> RATE_OF_REMAINING_DISTANCE_FOR_NEXT_BRAKING_/1, Unit_Delay4/1  "RATE_OF_REMAINING_DISTANCE_FOR_NEXT_BRAKING_"
  NEXT_ITERATION/1 -> Switch4/1  "NEXT_ITERATION"
  Unit_Delay4/1 -> Switch4/2, CAL__REMAINING_DISTANCE_FOR_NEXT_BRAKING_/1  "CAL__REMAINING_DISTANCE_FOR_NEXT_BRAKING_"

== system AEB_MODEL_F/AEB/AEB_SYSTEM/PARTIAL_BRAKE/PARTIAL_BRAKING/PB_IN_LOOP/SPEED ==
  note: ego_and_leading_vehicle_speed_comparison
  SPEED_AFTER_PARTITAL_BRAKE_ : Inport
  NEXT_ITERATION : Inport  Port=2
  Comp_speed_with_ego_vehicle : simulink/Logic and Bit Operations/Compare To Constant  relop=<=  const=SPEED_OF_THE_LEADING_VEHICLE  OutDataTypeStr=boolean
      settings: RTWMemSecFuncInitTerm=Inherit_from_model  RTWMemSecFuncExecute=Inherit_from_model  RTWMemSecDataConstants=Inherit_from_model  RTWMemSecDataInternal=Inherit_from_model  RTWMemSecDataParameters=Inherit_from_model
  Constant : Constant  Value=0
  Multiply : Gain  Gain=3.6
  Switch : Switch  Criteria=u2 > Threshold  SaturateOnIntegerOverflow=off  InputSameDT=off
  Switch4 : Switch  Criteria=u2 > Threshold  SaturateOnIntegerOverflow=off  InputSameDT=off
  Unit_Delay4 : UnitDelay  SampleTime=-1  HasFrameUpgradeWarning=on
  RATE_OF_SPEED : Outport
  CAL__SPEED_AFTER_PB_DECCELERATION : Outport  Port=2
  tag scope: comp_speed_ego_and_leading_pb=global
  wires:
  Unit_Delay4/1 -> Switch4/2, CAL__SPEED_AFTER_PB_DECCELERATION/1  "CAL__SPEED_AFTER_PB_DECCELERATION"
  SPEED_AFTER_PARTITAL_BRAKE_/1 -> Switch4/3  "SPEED_AFTER_PARTITAL_BRAKE_"
  NEXT_ITERATION/1 -> Switch4/1  "NEXT_ITERATION"
  Switch/1 -> RATE_OF_SPEED/1  "RATE_OF_SPEED"
  Comp_speed_with_ego_vehicle/1 -> Switch/2, [comp_speed_ego_and_leading_pb]
  Multiply/1 -> Comp_speed_with_ego_vehicle/1
  Constant/1 -> Switch/1
  Switch4/1 -> Unit_Delay4/1, Switch/3, Multiply/1

== system AEB_MODEL_F/AEB/AEB_SYSTEM/PARTIAL_BRAKE/PARTIAL_BRAKING/PB_IN_LOOP/TTC_AFTER_PARTIAL_BRAKING ==
  TTC_AFTER_PARTITAL_BRAKE : Inport
  NEXT_ITERATION : Inport  Port=2
  AND1 : Logic  IconShape=distinctive  AllPortsSameDT=off  OutDataTypeStr=boolean
  AND2 : Logic  IconShape=distinctive  AllPortsSameDT=off  OutDataTypeStr=boolean
  Compare_To_Constant1 : simulink/Logic and Bit Operations/Compare To Constant  relop=>=  const=0  OutDataTypeStr=boolean
      settings: RTWMemSecFuncInitTerm=Inherit_from_model  RTWMemSecFuncExecute=Inherit_from_model  RTWMemSecDataConstants=Inherit_from_model  RTWMemSecDataInternal=Inherit_from_model  RTWMemSecDataParameters=Inherit_from_model
  Compare_To_Constant2 : simulink/Logic and Bit Operations/Compare To Constant  relop=>=  const=0  OutDataTypeStr=boolean
      settings: RTWMemSecFuncInitTerm=Inherit_from_model  RTWMemSecFuncExecute=Inherit_from_model  RTWMemSecDataConstants=Inherit_from_model  RTWMemSecDataInternal=Inherit_from_model  RTWMemSecDataParameters=Inherit_from_model
  Compare_To_Constant3 : simulink/Logic and Bit Operations/Compare To Constant  relop===  const=0  OutDataTypeStr=boolean
      settings: RTWMemSecFuncInitTerm=Inherit_from_model  RTWMemSecFuncExecute=Inherit_from_model  RTWMemSecDataConstants=Inherit_from_model  RTWMemSecDataInternal=Inherit_from_model  RTWMemSecDataParameters=Inherit_from_model
  Compare_To_Constant4 : simulink/Logic and Bit Operations/Compare To Constant  relop=<=  const=0.01  OutDataTypeStr=boolean
      settings: RTWMemSecFuncInitTerm=Inherit_from_model  RTWMemSecFuncExecute=Inherit_from_model  RTWMemSecDataConstants=Inherit_from_model  RTWMemSecDataInternal=Inherit_from_model  RTWMemSecDataParameters=Inherit_from_model
  Constant : Constant  Value=0
  Constant1 : Constant  Value=0
  Switch1 : Switch  Criteria=u2 > Threshold  SaturateOnIntegerOverflow=off  InputSameDT=off
  Switch2 : Switch  Criteria=u2 > Threshold  SaturateOnIntegerOverflow=off  InputSameDT=off
  Switch4 : Switch  Criteria=u2 > Threshold  SaturateOnIntegerOverflow=off  InputSameDT=off
  Unit_Delay4 : UnitDelay  SampleTime=-1  HasFrameUpgradeWarning=on
  RATE_OF_TTC_AFTER_PARTITAL_BRAKE : Outport
  CAL__TTCmin : Outport  Port=2
  wires:
  Unit_Delay4/1 -> Switch4/2, CAL__TTCmin/1  "CAL__TTCmin"
  TTC_AFTER_PARTITAL_BRAKE/1 -> Switch4/3  "TTC_AFTER_PARTITAL_BRAKE"
  NEXT_ITERATION/1 -> Switch4/1  "NEXT_ITERATION"
  Compare_To_Constant2/1 -> AND1/1
  Compare_To_Constant3/1 -> AND1/2
  AND1/1 -> Switch1/2
  Switch1/1 -> Unit_Delay4/1
  Constant1/1 -> Switch1/1
  Switch2/1 -> RATE_OF_TTC_AFTER_PARTITAL_BRAKE/1  "RATE_OF_TTC_AFTER_PARTITAL_BRAKE"
  Switch4/1 -> Switch1/3, Compare_To_Constant3/1, Compare_To_Constant1/1, Switch2/3, Compare_To_Constant4/1, Compare_To_Constant2/1
  AND2/1 -> Switch2/2
  Constant/1 -> Switch2/1
  Compare_To_Constant1/1 -> AND2/1
  Compare_To_Constant4/1 -> AND2/2

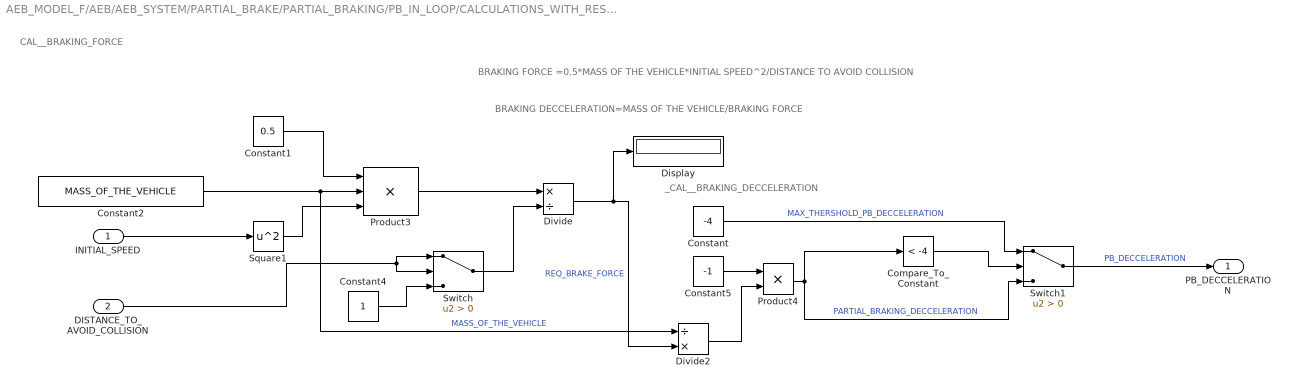
== system AEB_MODEL_F/AEB/AEB_SYSTEM/PARTIAL_BRAKE/PARTIAL_BRAKING/PB_IN_LOOP/CALCULATIONS_WITH_RESPECT_TO_TTC/CAL_BRAKING_DECCELERATION ==
  note: _CAL__BRAKING_DECCELERATION
  note: BRAKING DECCELERATION=MASS OF THE VEHICLE/BRAKING FORCE
  note: BRAKING FORCE =0.5*MASS OF THE VEHICLE*INITIAL SPEED^2/DISTANCE TO AVOID COLLISION
  note: CAL__BRAKING_FORCE
  INITIAL_SPEED : Inport
  DISTANCE_TO_AVOID_COLLISION : Inport  Port=2
  Compare_To_Constant : simulink/Logic and Bit Operations/Compare To Constant  relop=<  const=-4  OutDataTypeStr=boolean
      settings: RTWMemSecFuncInitTerm=Inherit_from_model  RTWMemSecFuncExecute=Inherit_from_model  RTWMemSecDataConstants=Inherit_from_model  RTWMemSecDataInternal=Inherit_from_model  RTWMemSecDataParameters=Inherit_from_model
  Constant : Constant  Value=-4
  Constant1 : Constant  Value=0.5
  Constant2 : Constant  Value=MASS_OF_THE_VEHICLE
  Constant4 : Constant
  Constant5 : Constant  Value=-1
  Display : Display
  Divide : Product  Inputs=*/
  Divide2 : Product  Inputs=/*
  Product3 : Product  Inputs=3
  Product4 : Product
  Square1 : Math  Operator=square
  Switch : Switch  Criteria=u2 > Threshold  SaturateOnIntegerOverflow=off  InputSameDT=off
  Switch1 : Switch  Criteria=u2 > Threshold  SaturateOnIntegerOverflow=off  InputSameDT=off
  PB_DECCELERATION : Outport
  wires:
  Divide2/1 -> Product4/2
  Switch1/1 -> PB_DECCELERATION/1  "PB_DECCELERATION"
  Constant2/1 -> Divide2/1, Product3/2  "MASS_OF_THE_VEHICLE"
  Constant5/1 -> Product4/1
  Switch/1 -> Divide/2
  Constant4/1 -> Switch/3
  Product4/1 -> Switch1/3, Compare_To_Constant/1  "PARTIAL_BRAKING_DECCELERATION"
  INITIAL_SPEED/1 -> Square1/1
  Constant1/1 -> Product3/1
  Product3/1 -> Divide/1
  DISTANCE_TO_AVOID_COLLISION/1 -> Switch/2, Switch/1
  Constant/1 -> Switch1/1  "MAX_THERSHOLD_PB_DECCELERATION"
  Divide/1 -> Display/1, Divide2/2  "REQ_BRAKE_FORCE"
  Compare_To_Constant/1 -> Switch1/2
  Square1/1 -> Product3/3

== system AEB_MODEL_F/AEB/AEB_SYSTEM/PARTIAL_BRAKE/PARTIAL_BRAKING/PB_IN_LOOP/CALCULATIONS_WITH_RESPECT_TO_TTC/CAL_TTC ==
  INITIAL_SPEED_M/S : Inport
  SPEED_AFTER_PB_DECCELERATION : Inport  Port=2
  Constant6 : Constant
  Divide1 : Product  Inputs=/*
  Switch2 : Switch  Criteria=u2 > Threshold  SaturateOnIntegerOverflow=off  InputSameDT=off
  TTC_AFTER_PARTITAL_BRAKE : Outport
  wires:
  Constant6/1 -> Switch2/3
  Switch2/1 -> Divide1/1
  INITIAL_SPEED_M/S/1 -> Switch2/2, Switch2/1  "INITIAL_SPEED_M/S"
  SPEED_AFTER_PB_DECCELERATION/1 -> Divide1/2  "SPEED_AFTER_PB_DECCELERATION"
  Divide1/1 -> TTC_AFTER_PARTITAL_BRAKE/1  "TTC_AFTER_PARTITAL_BRAKE"

== system AEB_MODEL_F/AEB/AEB_SYSTEM/PARTIAL_BRAKE/PARTIAL_BRAKING/PB_IN_LOOP/CALCULATIONS_WITH_RESPECT_TO_TTC/CAL_inital_after_decceleration_speed ==
  note: Speed_after_deceleration:V=u+at
  INITIAL_SPEED : Inport
  TTC_PB : Inport  Port=2
  PARTIAL_BRAKING_DECCELERATION : Inport  Port=3
  Product5 : Product
  Subtract1 : Sum
  INITIAL_SPEED_M/S : Outport
  SPEED_AFTER_PB_DECCELERATION : Outport  Port=2
  wires:
  INITIAL_SPEED/1 -> Subtract1/1  "INITIAL_SPEED"
  PARTIAL_BRAKING_DECCELERATION/1 -> Product5/1  "PARTIAL_BRAKING_DECCELERATION"
  Product5/1 -> Subtract1/2
  Subtract1/1 -> SPEED_AFTER_PB_DECCELERATION/1, INITIAL_SPEED_M/S/1  "INITIAL_SPEED"
  TTC_PB/1 -> Product5/2  "TTC_PB"

== system AEB_MODEL_F/AEB/AEB_SYSTEM/PARTIAL_BRAKE/PARTIAL_BRAKING/PB_IN_LOOP/CALCULATIONS_WITH_RESPECT_TO_TTC/CAL_remainig_distance ==
  note: Remaining distance= ut + 1/2(at^2)
  INITIAL_SPEED : Inport
  DISTANCE_TO_AVOID_COLLISION : Inport  Port=2
  TTC_PB : Inport  Port=3
  PB_DECCELERATION : Inport  Port=4
  Add1 : Sum
  Constant3 : Constant  Value=0.5
  Product1 : Product  Inputs=3
  Product2 : Product
  Square2 : Math  Operator=square
  Subtract3 : Sum  Inputs=+-
  Remainig_distance : Outport
  wires:
  Add1/1 -> Subtract3/2
  TTC_PB/1 -> Square2/1, Product2/2  "TTC_PB"
  Square2/1 -> Product1/3
  Subtract3/1 -> Remainig_distance/1  "Remainig_distance"
  Product1/1 -> Add1/2
  Product2/1 -> Add1/1
  Constant3/1 -> Product1/1
  PB_DECCELERATION/1 -> Product1/2  "PB_DECCELERATION"
  DISTANCE_TO_AVOID_COLLISION/1 -> Subtract3/1  "DISTANCE_TO_AVOID_COLLISION"
  INITIAL_SPEED/1 -> Product2/1  "INITIAL_SPEED"

== system AEB_MODEL_F/AEB/AEB_SYSTEM/PARTIAL_BRAKE/PARTIAL_BRAKING/PB_IN_LOOP/CALCULATIONS_WITH_RESPECT_TO_TTC/TTC_LIMIT ==
  TTC_PB_ : Inport
  AND1 : Logic  IconShape=distinctive  AllPortsSameDT=off  OutDataTypeStr=boolean
  Compare_To_Constant2 : simulink/Logic and Bit Operations/Compare To Constant  relop=<=  const=0.03  OutDataTypeStr=boolean
      settings: RTWMemSecFuncInitTerm=Inherit_from_model  RTWMemSecFuncExecute=Inherit_from_model  RTWMemSecDataConstants=Inherit_from_model  RTWMemSecDataInternal=Inherit_from_model  RTWMemSecDataParameters=Inherit_from_model
  Compare_To_Constant3 : simulink/Logic and Bit Operations/Compare To Constant  relop=>  const=0  OutDataTypeStr=boolean
      settings: RTWMemSecFuncInitTerm=Inherit_from_model  RTWMemSecFuncExecute=Inherit_from_model  RTWMemSecDataConstants=Inherit_from_model  RTWMemSecDataInternal=Inherit_from_model  RTWMemSecDataParameters=Inherit_from_model
  Constant : Constant  Value=0
  Switch1 : Switch  Criteria=u2 > Threshold  SaturateOnIntegerOverflow=off  InputSameDT=off
  TTC_PB : Outport
  wires:
  AND1/1 -> Switch1/2
  Compare_To_Constant3/1 -> AND1/2
  Compare_To_Constant2/1 -> AND1/1
  TTC_PB_/1 -> Compare_To_Constant2/1, Switch1/3, Compare_To_Constant3/1
  Switch1/1 -> TTC_PB/1
  Constant/1 -> Switch1/1
